simulink model "basicBehavior"  (R2023a)
settings: Solver=FixedStepAuto  StartTime=0.0  StopTime=2000  RelTol=1e-3
undefined symbols (not defined in the file or in its folder): Ended, Single
libraries: speedgoatlib_IO191 x2
settings Model: Creator=electro  LastModifiedBy=electro
settings SolverCC: ConcurrentTasks=on  PositivePriorityOrder=on  AutoInsertRateTranBlk=on
settings OptimizationCC: BlockReduction=off  OptimizeBlockIOStorage=off  EnhancedBackFolding=on  PassReuseOutputArgsThreshold=0  OptimizeBlockOrder=speed  DifferentSizesBufferReuse=on
settings DebuggingCC: TasksWithSamePriorityMsg=none  ParameterTunabilityLossMsg=error  SFUnexpectedBacktrackingDiag=warning  SFNoUnconditionalDefaultTransitionDiag=warning
settings HardwareCC: ProdBitPerLong=64  ProdLongLongMode=on  ProdHWDeviceType=Intel->x86-64 (Linux 64)
settings SFSimCC: SimUserIncludeDirs="\"/usr/local/MATLAB/R2023a/toolbox/slrealtime/target/kernel/dist/include/verify\""  MATLABDynamicMemAlloc=off
settings RTWCC: Description=Simulink Real-Time  SystemTargetFile=slrealtime.tlc  TemplateMakefile=slrealtime_default_tmf  GenerateReport=on  RTWVerbose=off  CustomInclude=/usr/local/MATLAB/R2023a/toolbox/slrealtime/target/kernel/dist/include,  Toolchain=Simulink Real-Time Toolchain  BuildConfiguration=Faster Runs  CodeExecutionProfiling=on  TargetLang=C++
settings CodeAppCC: ForceParamTrailComments=on  OperatorAnnotations=on  EnableCustomComments=on

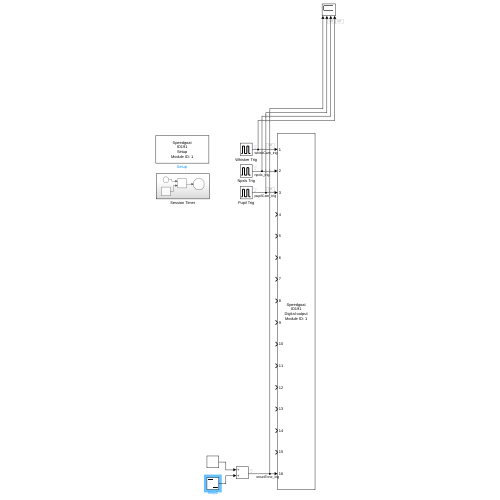
[thumbnail: Simulink's stored preview of the top-level diagram]
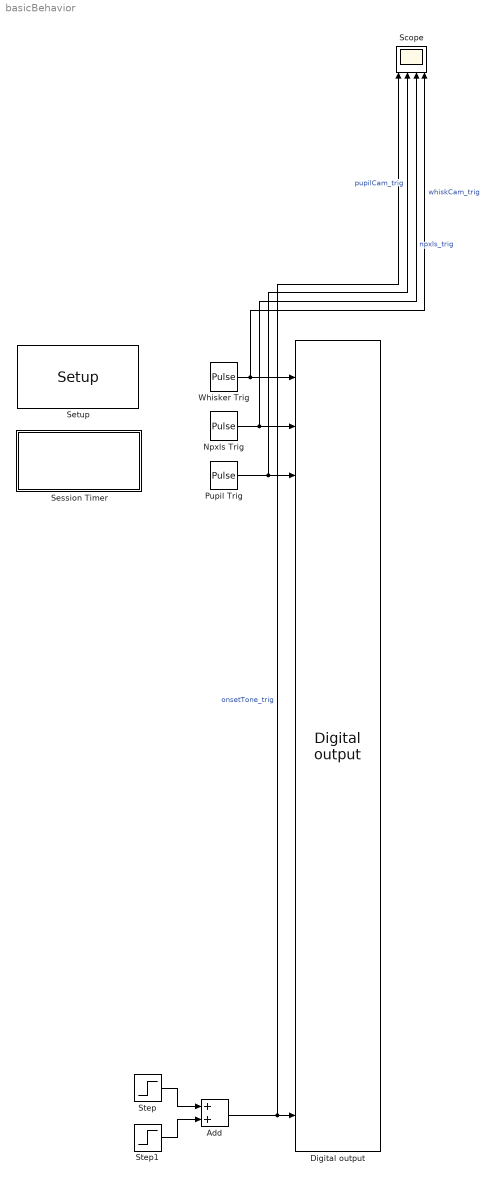
== system basicBehavior ==
  Add : Sum
  "Digital output " : speedgoatlib_IO191/Digital output   parModuleId=1  parSampleTime=0.002  parPciSlot=-1  parDoChannels=[1 2 3 4 5 6 7 8 9 10 11 12 13 14 15 16]  parDoInitValues=[0 0 0 0 0 0 0 0 0 0 0 0 0 0 0 0]  parDoResets=[1 1 1 1 1 1 1 1 1 1 1 1 1 1 1 1]
      settings: SourceProductName=Simulink Real-Time: Speedgoat I/O Blockset
  Npxls Trig : DiscretePulseGenerator  PulseType=Time based  Period=0.004  PulseWidth=50  SampleTime=0.002
  Pupil Trig : DiscretePulseGenerator  PulseType=Time based  Period=0.1  PulseWidth=50  SampleTime=0.002
  Scope : Scope  NumInputPorts=4
  Session Timer : Subsystem
  "Setup " : speedgoatlib_IO191/Setup   parModuleId=1  parPciSlot=-1  parTriggerSignal=TTL  parAdcChannels=[1 2]  parAdcRanges=[3 3]  parAdcChannel1=on  parAdcChannel2=on  parAdcChannel3=off  parAdcChannel4=off  parAdcChannel5=off  parAdcChannel6=off  parAdcChannel7=off  parAdcChannel8=off  parAdcMode=Single-Ended  parAdcRate=100000  parAdcRange11=+-10.24 V  parAdcRange21=+-24.576 V  parAdcRange12=+-10.24 V  parAdcRange22=+-24.576 V  parAdcRange13=+-10.24 V  parAdcRange23=+-24.576 V  parAdcRange14=+-10.24 V  parAdcRange24=+-24.576 V  parAdcRange15=+-10.24 V  parAdcRange25=+-24.576 V  parAdcRange16=+-10.24 V  parAdcRange26=+-24.576 V  parAdcRange17=+-10.24 V  parAdcRange27=+-24.576 V  parAdcRange18=+-10.24 V  parAdcRange28=+-24.576 V  parDacChannels=[1 2]  parDacChannel1=on  parDacChannel2=on  parDacChannel3=off  parDacChannel4=off  parDacMode=Single-Ended  parDacRanges=[4 4]  parDacInitValues=[0 0]  parDacResets=[1 1]  parDacRange1=+-10 V  parDacInitValue1=0  parDacReset1=on  parDacRange2=+-10 V  parDacInitValue2=0  parDacReset2=on  parDacRange3=+-10 V  parDacInitValue3=0  parDacReset3=on  parDacRange4=+-10 V  parDacInitValue4=0  parDacReset4=on  parDiChannels=zeros(1,0)  parDoChannels=[1 2 3 4 5 6 7 8 9 10 11 12 13 14 15 16]  parDioFirstControl=[1 2 3 4 5 6 7 8 9]  parDioSecondControl=0  parDioChannel1=Out  parExtra1=I  parExtra2=I  parExtra3=I  parDioChannel2=Out  parDioChannel3=Out  parDioChannel4=Out  parDioChannel5=Out  parDioChannel6=Out  parDioChannel7=Out  parDioChannel8=Out  parDioChannel9=Out  parDoInitValues=[0 0 0 0]  parDoResets=[1 1 1 1]  parDoInitValue1=0  parDoReset1=on  parDoInitValue2=0  parDoReset2=on  parDoInitValue3=0  parDoReset3=on  parDoInitValue4=0  parDoReset4=on  parDoInitValue5=0  parDoReset5=on  parDoInitValue6=0  parDoReset6=on  parDoInitValue7=0  parDoReset7=on  parDoInitValue8=0  parDoReset8=on  parDoInitValue9=0  parDoReset9=on  parDoInitValue10=0  parDoReset10=on  parDoInitValue11=0  parDoReset11=on  parDoInitValue12=0  parDoReset12=on  parDoInitValue13=0  parDoReset13=on  parDoInitValue14=0  parDoReset14=on  parDoInitValue15=0  parDoReset15=on  parDoInitValue16=0  parDoReset16=on
      settings: SourceProductName=Simulink Real-Time: Speedgoat I/O Blockset
  Step : Step  Time=0  SampleTime=0.002
  Step1 : Step  After=-1  SampleTime=0.002
  Whisker Trig : DiscretePulseGenerator  PulseType=Time based  Period=0.02  PulseWidth=50  SampleTime=0.002
  wires:
  Whisker Trig/1 -> Scope/4, "Digital output "/1  "whiskCam_trig"
  Pupil Trig/1 -> Scope/2, "Digital output "/3  "pupilCam_trig"
  Add/1 -> Scope/1, "Digital output "/16  "onsetTone_trig"
  Npxls Trig/1 -> Scope/3, "Digital output "/2  "npxls_trig"
  Step/1 -> Add/1
  Step1/1 -> Add/2

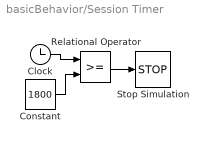
== system basicBehavior/Session Timer ==
  Clock : Clock
  Constant : Constant  Value=1800  SampleTime=0.002
  Relational Operator : RelationalOperator  OutDataTypeStr=boolean  RndMeth=Simplest  InputSameDT=off
  Stop Simulation : Stop
  wires:
  Relational Operator/1 -> Stop Simulation/1
  Constant/1 -> Relational Operator/2
  Clock/1 -> Relational Operator/1
